simulink model "examples_of_mux_block"  (R2021a)
settings: Solver=VariableStepAuto  StartTime=0.0  StopTime=1  RelTol=1e-3
settings Model: Creator=YasserNet  LastModifiedBy=YasserNet

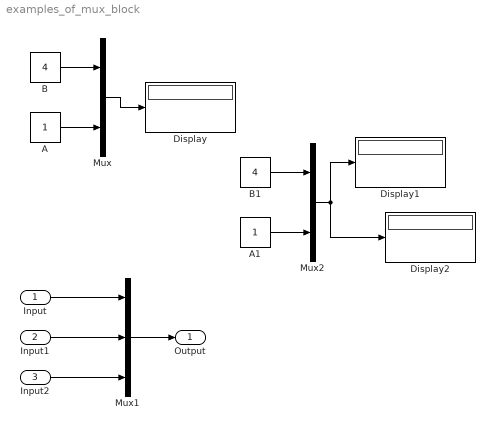
== system examples_of_mux_block ==
  Input : Inport
  Input1 : Inport  Port=2
  Input2 : Inport  Port=3
  A : Constant
  A1 : Constant
  B : Constant  Value=4
  B1 : Constant  Value=4
  Display : Display
  Display1 : Display
  Display2 : Display
  Mux : Mux  Inputs=2
  Mux1 : Mux  Inputs=3
  Mux2 : Mux  Inputs=2
  Output : Outport
  wires:
  Mux/1 -> Display/1
  B/1 -> Mux/1
  A/1 -> Mux/2
  Input2/1 -> Mux1/3
  Input/1 -> Mux1/1
  Input1/1 -> Mux1/2
  Mux1/1 -> Output/1
  A1/1 -> Mux2/2
  B1/1 -> Mux2/1
  Mux2/1 -> Display2/1, Display1/1
